simulink model "Main_Sim"  (R2018b)
settings: Solver=FixedStepAuto  StartTime=0.0  StopTime=10800  FixedStep=simParams.sample_time_s  RelTol=1e-3  EnableMultiTasking=on
values from neighbouring files (symbols this model uses):
  test_data = struct    [Sim_init.m]
undefined symbols (not defined in the file or in its folder): actuators_lib, Actuators_Lib, FSW_Lib, gyro_body_radps, gyro_meas_valid, mag_body_T, mag_meas_valid, photodiodes_A, simParams, solar_panel_power_W, sunsensor_body_deg, sunsensor_valid
libraries: gyroscope_lib x3, magnetometer_lib x3, dspstat3 x2, simulink_extras x2, rwa_assembly_torqueinput_lib x1, Environment_lib x1, allocation_lib x1, control_command_generation_lib x1, mode_select_lib x1, target_gen_lib x1, solar_panels_lib x1, sun_sensor_lib x1
settings Model: Creator=devantormey  LastModifiedBy=jeric
settings OptimizationCC: LifeSpan=inf
settings DebuggingCC: SFUnexpectedBacktrackingDiag=warning  SFNoUnconditionalDefaultTransitionDiag=warning
settings SFSimCC: SimUseLocalCustomCode=off
settings RTWCC: RTWUseLocalCustomCode=off
settings CodeAppCC: StateflowObjectComments=on
settings GRTTargetCC: TargetLangStandard=C89/C90 (ANSI)  GeneratePreprocessorConditionals=Disable all
settings ConfigComp: CovMetricSettings=dw  CovHtmlReporting=on  CovSaveCumulativeToWorkspaceVar=on  CovSaveSingleToWorkspaceVar=on  CovExternalEMLEnable=off

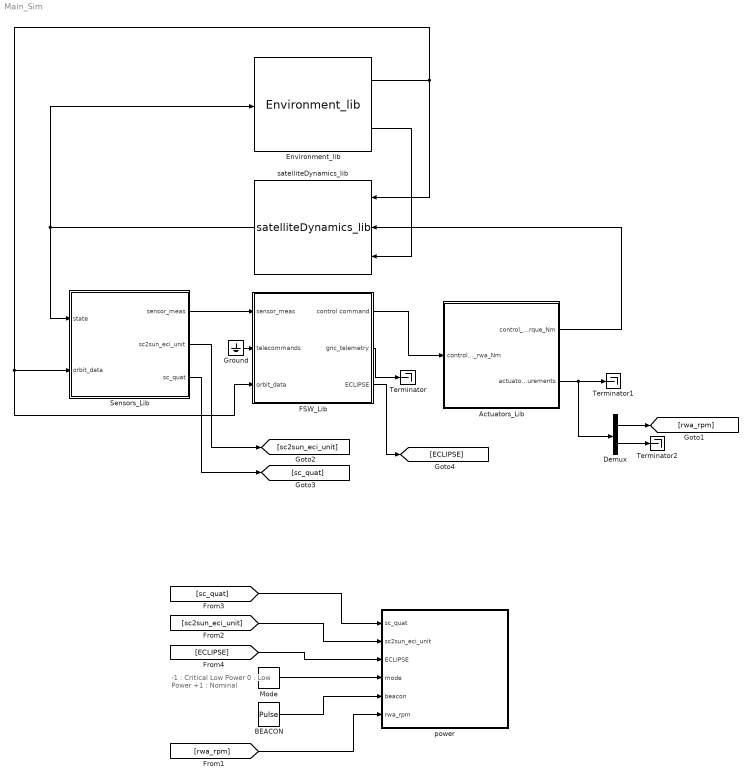
== system Main_Sim ==
  note: -1	: Critical Low Power
      |   0	: Low Power
      | +1	: Nominal
  Actuators_Lib : Subsystem  AncestorBlock=actuators_lib/Actuators_Lib
  BEACON : DiscretePulseGenerator  PulseType=Time based  Period=60  PulseWidth=100 * (1.0 / 60)
  Demux : Demux  Outputs=[4 4]
  Environment_lib : Environment_lib/Environment_lib  SystemSampleTime=-1
  FSW_Lib : Subsystem  AncestorBlock=FSW_Lib/FSW_Lib
  Ground : Ground
  Mode : Constant
  Sensors_Lib : Subsystem
  Terminator : Terminator
  Terminator1 : Terminator
  Terminator2 : Terminator
  power : Subsystem
  satelliteDynamics_lib : satelliteDynamics_lib/satelliteDynamics_lib  SystemSampleTime=-1
  wires:
  FSW_Lib/1(control command) -> Actuators_Lib/1(control_cmd_rwa_Nm)
  Sensors_Lib/1(sensor_meas) -> FSW_Lib/1(sensor_meas)
  satelliteDynamics_lib/1 -> Environment_lib/1, Sensors_Lib/1(state)
  Environment_lib/1 -> FSW_Lib/3(orbit_data), Sensors_Lib/2(orbit_data), satelliteDynamics_lib/1
  Environment_lib/2 -> satelliteDynamics_lib/3
  Actuators_Lib/1(control_torque_Nm) -> satelliteDynamics_lib/2
  Ground/1 -> FSW_Lib/2(telecommands)
  FSW_Lib/2(gnc_telemetry) -> Terminator/1
  Actuators_Lib/2(actuator_measurements) -> Demux/1, Terminator1/1
  Demux/1 -> [rwa_rpm]
  Demux/2 -> Terminator2/1
  Sensors_Lib/2(sc2sun_eci_unit) -> [sc2sun_eci_unit]
  Sensors_Lib/3(sc_quat) -> [sc_quat]
  FSW_Lib/3(ECLIPSE) -> [ECLIPSE]
  [sc2sun_eci_unit] -> power/2(sc2sun_eci_unit)
  [sc_quat] -> power/1(sc_quat)
  [ECLIPSE] -> power/3(ECLIPSE)
  Mode/1 -> power/4(mode)
  BEACON/1 -> power/5(beacon)
  [rwa_rpm] -> power/6(rwa_rpm)

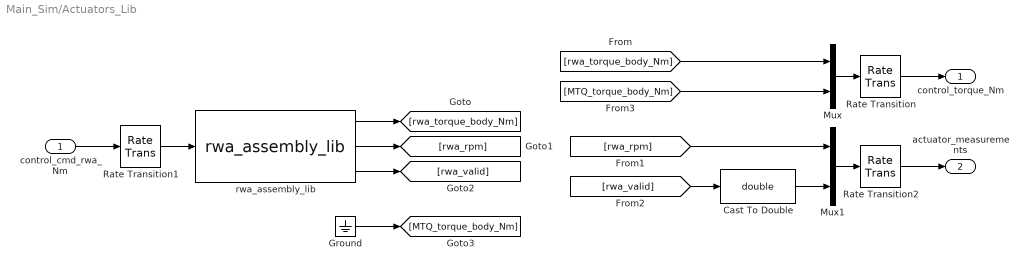
== system Main_Sim/Actuators_Lib ==
  control_cmd_rwa_Nm : Inport
  Cast To Double : DataTypeConversion  OutDataTypeStr=double
  Ground : Ground
  Mux : Mux  Inputs=[3 3]
  Mux1 : Mux  Inputs=[4 4]
  Rate Transition : RateTransition
  Rate Transition1 : RateTransition  OutPortSampleTimeOpt=Inherit  OutPortSampleTime=simParams.actuators.sample_time_s
  Rate Transition2 : RateTransition
  rwa_assembly_lib : rwa_assembly_torqueinput_lib/rwa_assembly_lib  SystemSampleTime=-1
  control_torque_Nm : Outport
  actuator_measurements : Outport  Port=2
  wires:
  Cast To Double/1 -> Mux1/2
  Rate Transition2/1 -> actuator_measurements/1
  Ground/1 -> [MTQ_torque_body_Nm]
  Mux/1 -> Rate Transition/1
  [rwa_torque_body_Nm] -> Mux/1
  [MTQ_torque_body_Nm] -> Mux/2
  Rate Transition1/1 -> rwa_assembly_lib/1
  Mux1/1 -> Rate Transition2/1
  [rwa_valid] -> Cast To Double/1
  [rwa_rpm] -> Mux1/1
  rwa_assembly_lib/1 -> [rwa_torque_body_Nm]
  rwa_assembly_lib/3 -> [rwa_valid]
  rwa_assembly_lib/2 -> [rwa_rpm]
  control_cmd_rwa_Nm/1 -> Rate Transition1/1
  Rate Transition/1 -> control_torque_Nm/1

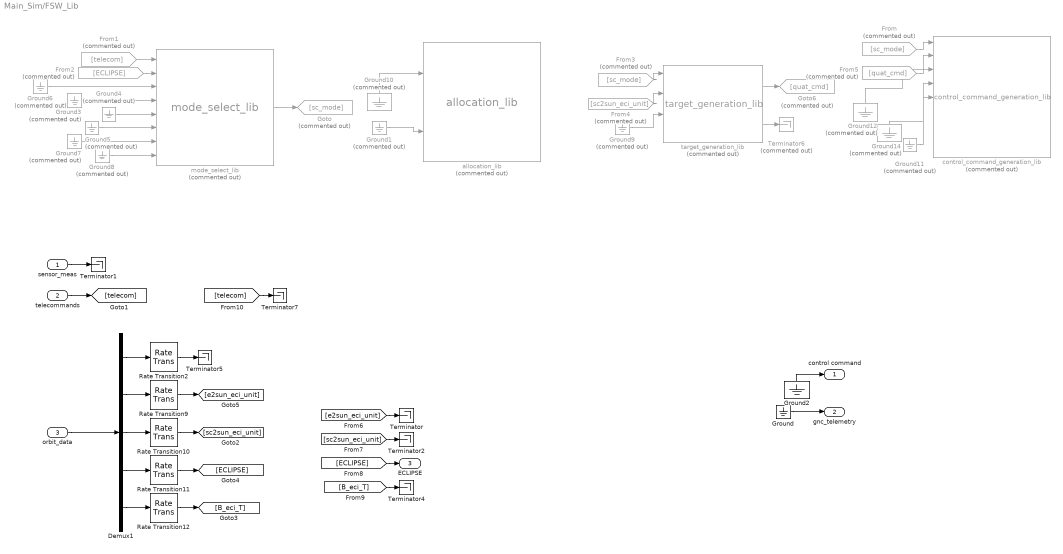
== system Main_Sim/FSW_Lib ==
  sensor_meas : Inport
  telecommands : Inport  Port=2
  orbit_data : Inport  Port=3
  Demux1 : Demux  Outputs=[3 3 3 1 3]
  From : From  Commented=on  GotoTag=sc_mode
  From1 : From  Commented=on  GotoTag=telecom
  From2 : From  Commented=on  GotoTag=ECLIPSE
  From3 : From  Commented=on  GotoTag=sc_mode
  From4 : From  Commented=on  GotoTag=sc2sun_eci_unit
  From5 : From  Commented=on  GotoTag=quat_cmd
  Goto : Goto  Commented=on  GotoTag=sc_mode
  Goto6 : Goto  Commented=on  GotoTag=quat_cmd
  Ground : Ground
  Ground{1,3..12,14} (12 alike) : Ground  Commented=on
  Ground2 : Ground
  Rate Transition{2,9..12} (5 alike) : RateTransition  OutPortSampleTime=simParams.sensors.sample_time_s
  Terminator{,1..2,4..5,7} (6 alike) : Terminator
  Terminator6 : Terminator  Commented=on
  allocation_lib : allocation_lib/allocation_lib  Commented=on  SystemSampleTime=-1
  control_command_generation_lib : control_command_generation_lib/control_command_generation_lib  Commented=on  SystemSampleTime=-1
  mode_select_lib : mode_select_lib/mode_select_lib  Commented=on  SystemSampleTime=-1
  target_generation_lib : target_gen_lib/target_generation_lib  Commented=on  SystemSampleTime=-1
  control command : Outport
  gnc_telemetry : Outport  Port=2
  ECLIPSE : Outport  Port=3
  wires:
  [telecom] -> Terminator7/1
  [B_eci_T] -> Terminator4/1
  [ECLIPSE] -> ECLIPSE/1
  [sc2sun_eci_unit] -> Terminator2/1
  [e2sun_eci_unit] -> Terminator/1
  Ground14/1 -> control_command_generation_lib/4
  Ground11/1 -> control_command_generation_lib/5
  Ground12/1 -> control_command_generation_lib/3
  Ground1/1 -> allocation_lib/2
  Ground10/1 -> allocation_lib/1
  From5/1 -> control_command_generation_lib/2
  Ground9/1 -> target_generation_lib/3
  target_generation_lib/1 -> Goto6/1
  target_generation_lib/2 -> Terminator6/1
  From4/1 -> target_generation_lib/2
  From3/1 -> target_generation_lib/1
  Ground8/1 -> mode_select_lib/8
  Ground7/1 -> mode_select_lib/7
  Ground6/1 -> mode_select_lib/3
  Ground5/1 -> mode_select_lib/6
  Ground4/1 -> mode_select_lib/5
  Ground3/1 -> mode_select_lib/4
  From2/1 -> mode_select_lib/2
  Demux1/4 -> Rate Transition11/1
  Rate Transition2/1 -> Terminator5/1
  Demux1/5 -> Rate Transition12/1
  Rate Transition9/1 -> [e2sun_eci_unit]
  Rate Transition10/1 -> [sc2sun_eci_unit]
  Demux1/3 -> Rate Transition10/1
  Rate Transition12/1 -> [B_eci_T]
  Demux1/1 -> Rate Transition2/1
  Rate Transition11/1 -> [ECLIPSE]
  Demux1/2 -> Rate Transition9/1
  orbit_data/1 -> Demux1/1
  From1/1 -> mode_select_lib/1
  From/1 -> control_command_generation_lib/1
  mode_select_lib/1 -> Goto/1
  Ground2/1 -> control command/1
  Ground/1 -> gnc_telemetry/1
  telecommands/1 -> [telecom]
  sensor_meas/1 -> Terminator1/1

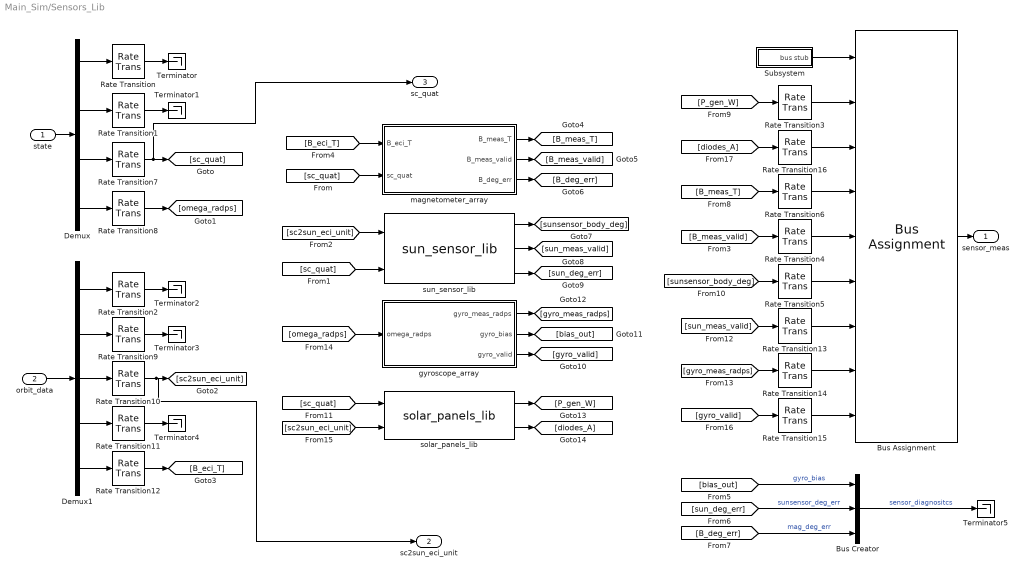
== system Main_Sim/Sensors_Lib ==
  state : Inport
  orbit_data : Inport  Port=2
  Bus Assignment : BusAssignment  AssignedSignals=solar_panel_power_W,photodiodes_A,mag_body_T,mag_meas_valid,sunsensor_body_deg,sunsensor_valid,gyro_body_radps,gyro_meas_valid
  Bus Creator : BusCreator  Inputs=3
  Demux : Demux  Outputs=[3 3 4 3]
  Demux1 : Demux  Outputs=[3 3 3 1 3]
  Rate Transition{,1..16} (17 alike) : RateTransition  OutPortSampleTime=simParams.sensors.sample_time_s
  Subsystem : Subsystem
  Terminator{,1..5} (6 alike) : Terminator
  gyroscope_array : Subsystem
  magnetometer_array : Subsystem
  solar_panels_lib : solar_panels_lib/solar_panels_lib  SystemSampleTime=-1
  "sun_sensor_lib " : sun_sensor_lib/sun_sensor_lib   SystemSampleTime=-1
  sensor_meas : Outport
  sc2sun_eci_unit : Outport  Port=2
  sc_quat : Outport  Port=3
  wires:
  [diodes_A] -> Rate Transition16/1
  Rate Transition16/1 -> Bus Assignment/3
  Rate Transition3/1 -> Bus Assignment/2
  Rate Transition6/1 -> Bus Assignment/4
  Rate Transition4/1 -> Bus Assignment/5
  Rate Transition5/1 -> Bus Assignment/6
  Rate Transition13/1 -> Bus Assignment/7
  Rate Transition14/1 -> Bus Assignment/8
  Rate Transition15/1 -> Bus Assignment/9
  solar_panels_lib/2 -> [diodes_A]
  Bus Creator/1 -> Terminator5/1  "sensor_diagnositcs"
  [B_deg_err] -> Bus Creator/3  "mag_deg_err"
  [sun_deg_err] -> Bus Creator/2  "sunsensor_deg_err"
  [bias_out] -> Bus Creator/1  "gyro_bias"
  [gyro_valid] -> Rate Transition15/1
  [gyro_meas_radps] -> Rate Transition14/1
  [sun_meas_valid] -> Rate Transition13/1
  [sunsensor_body_deg] -> Rate Transition5/1
  [B_meas_valid] -> Rate Transition4/1
  [P_gen_W] -> Rate Transition3/1
  [B_meas_T] -> Rate Transition6/1
  solar_panels_lib/1 -> [P_gen_W]
  [sc_quat] -> solar_panels_lib/1
  [sc2sun_eci_unit] -> solar_panels_lib/2
  Demux1/1 -> Rate Transition2/1
  Rate Transition2/1 -> Terminator2/1
  Rate Transition9/1 -> Terminator3/1
  Demux1/2 -> Rate Transition9/1
  Rate Transition10/1 -> sc2sun_eci_unit/1, [sc2sun_eci_unit]
  Demux1/3 -> Rate Transition10/1
  Rate Transition11/1 -> Terminator4/1
  Demux1/4 -> Rate Transition11/1
  Rate Transition12/1 -> [B_eci_T]
  Demux1/5 -> Rate Transition12/1
  Rate Transition/1 -> Terminator/1
  Demux/1 -> Rate Transition/1
  Rate Transition1/1 -> Terminator1/1
  Demux/2 -> Rate Transition1/1
  Rate Transition7/1 -> sc_quat/1, [sc_quat]
  Demux/3 -> Rate Transition7/1
  Demux/4 -> Rate Transition8/1
  Rate Transition8/1 -> [omega_radps]
  gyroscope_array/3(gyro_valid) -> [gyro_valid]
  gyroscope_array/2(gyro_bias) -> [bias_out]
  gyroscope_array/1(gyro_meas_radps) -> [gyro_meas_radps]
  "sun_sensor_lib "/3 -> [sun_deg_err]
  "sun_sensor_lib "/2 -> [sun_meas_valid]
  "sun_sensor_lib "/1 -> [sunsensor_body_deg]
  magnetometer_array/3(B_deg_err) -> [B_deg_err]
  magnetometer_array/2(B_meas_valid) -> [B_meas_valid]
  magnetometer_array/1(B_meas_T) -> [B_meas_T]
  Subsystem/1(bus stub) -> Bus Assignment/1
  [B_eci_T] -> magnetometer_array/1(B_eci_T)
  [sc2sun_eci_unit] -> "sun_sensor_lib "/1
  orbit_data/1 -> Demux1/1
  [omega_radps] -> gyroscope_array/1(omega_radps)
  [sc_quat] -> "sun_sensor_lib "/2
  [sc_quat] -> magnetometer_array/2(sc_quat)
  state/1 -> Demux/1
  Bus Assignment/1 -> sensor_meas/1

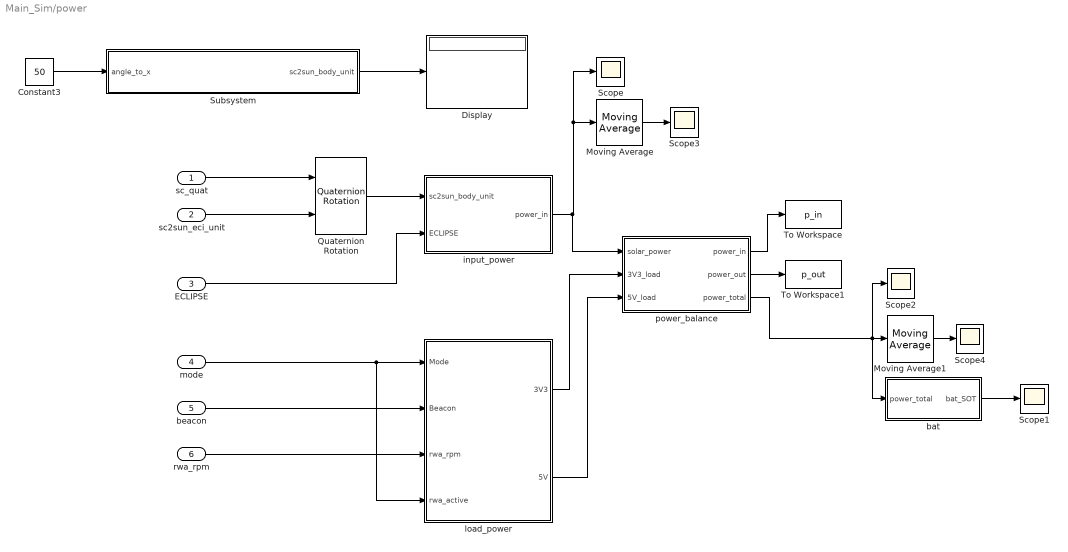
== system Main_Sim/power ==
  sc_quat : Inport
  sc2sun_eci_unit : Inport  Port=2
  ECLIPSE : Inport  Port=3
  mode : Inport  Port=4
  beacon : Inport  Port=5
  rwa_rpm : Inport  Port=6
  Constant3 : Constant  Value=50
  Display : Display
  Moving Average : dspstat3/Moving Average  Method=Exponential weighting  ForgettingFactorPort=off  SpecifyWindowLength=on  WindowLength=4  ForgettingFactor=1.0  SimulateUsing=Code generation
  Moving Average1 : dspstat3/Moving Average  Method=Exponential weighting  ForgettingFactorPort=off  SpecifyWindowLength=on  WindowLength=4  ForgettingFactor=1.0  SimulateUsing=Code generation
  Quaternion Rotation : aerolibutil/Quaternion Rotation
  Scope{,1..4} (5 alike) : Scope
  Subsystem : Subsystem
  To Workspace : ToWorkspace  VariableName=p_in  SampleTime=-1
  To Workspace1 : ToWorkspace  VariableName=p_out  SampleTime=-1
  bat : Subsystem
  input_power : Subsystem
  load_power : Subsystem
  power_balance : Subsystem
  wires:
  load_power/1(3V3) -> power_balance/2("3V3_load ")
  input_power/1(power_in) -> power_balance/1(solar_power), Moving Average/1, Scope/1
  rwa_rpm/1 -> load_power/3(rwa_rpm)
  mode/1 -> load_power/4(rwa_active), load_power/1(Mode)
  beacon/1 -> load_power/2(Beacon)
  Moving Average1/1 -> Scope4/1
  load_power/2(5V) -> power_balance/3(5V_load)
  bat/1(bat_SOT) -> Scope1/1
  Moving Average/1 -> Scope3/1
  sc_quat/1 -> Quaternion Rotation/1
  sc2sun_eci_unit/1 -> Quaternion Rotation/2
  ECLIPSE/1 -> input_power/2(ECLIPSE)
  power_balance/3(power_total) -> Scope2/1, bat/1(power_total), Moving Average1/1
  power_balance/1(power_in) -> To Workspace/1
  power_balance/2(power_out) -> To Workspace1/1
  Constant3/1 -> Subsystem/1(angle_to_x)
  Subsystem/1(sc2sun_body_unit) -> Display/1
  Quaternion Rotation/1 -> input_power/1(sc2sun_body_unit)

== system Main_Sim/Sensors_Lib/Subsystem ==
  Bus Creator : BusCreator  Inputs=8
  Constant : Constant  Value=zeros(6, 1)
  Constant1 : Constant  Value=zeros(3, simParams.sensors.mag.N_mag)
  Constant2 : Constant  Value=zeros(2, 1)
  Constant3 : Constant  Value=zeros(3, simParams.sensors.gyro.N_gyro)
  Constant4 : Constant  Value=zeros(1,simParams.sensors.mag.N_mag)
  Constant5 : Constant  Value=0
  Constant6 : Constant  Value=zeros(1,simParams.sensors.gyro.N_gyro)
  Constant7 : Constant  Value=zeros(6, 1)
  bus stub : Outport
  wires:
  Constant7/1 -> Bus Creator/2  "photodiodes_A"
  Constant6/1 -> Bus Creator/8  "gyro_meas_valid"
  Constant5/1 -> Bus Creator/6  "sunsensor_valid"
  Constant4/1 -> Bus Creator/4  "mag_meas_valid"
  Constant3/1 -> Bus Creator/7  "gyro_body_radps"
  Bus Creator/1 -> bus stub/1
  Constant2/1 -> Bus Creator/5  "sunsensor_body_deg"
  Constant1/1 -> Bus Creator/3  "mag_body_T"
  Constant/1 -> Bus Creator/1  "solar_panel_power_W"

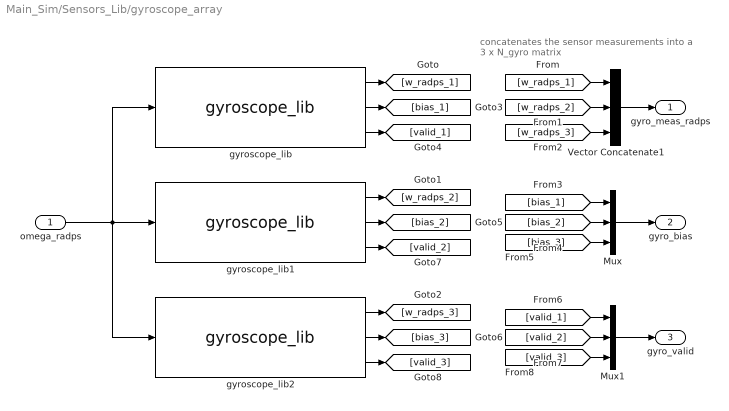
== system Main_Sim/Sensors_Lib/gyroscope_array ==
  note: concatenates the sensor measurements
      | into a 3 x N_gyro matrix
  omega_radps : Inport
  Mux : Mux  Inputs=3
  Mux1 : Mux  Inputs=3
  Vector Concatenate1 : Concatenate  NumInputs=3  Mode=Multidimensional array  ConcatenateDimension=2
  gyroscope_lib : gyroscope_lib/gyroscope_lib  id_s=1
  gyroscope_lib1 : gyroscope_lib/gyroscope_lib  id_s=2
  gyroscope_lib2 : gyroscope_lib/gyroscope_lib  id_s=3
  gyro_meas_radps : Outport
  gyro_bias : Outport  Port=2
  gyro_valid : Outport  Port=3
  wires:
  [valid_3] -> Mux1/3
  [valid_2] -> Mux1/2
  [valid_1] -> Mux1/1
  Mux1/1 -> gyro_valid/1
  [bias_3] -> Mux/3
  [bias_2] -> Mux/2
  [bias_1] -> Mux/1
  Mux/1 -> gyro_bias/1
  [w_radps_3] -> Vector Concatenate1/3
  [w_radps_2] -> Vector Concatenate1/2
  [w_radps_1] -> Vector Concatenate1/1
  Vector Concatenate1/1 -> gyro_meas_radps/1
  gyroscope_lib2/3 -> [valid_3]
  gyroscope_lib1/3 -> [valid_2]
  gyroscope_lib2/2 -> [bias_3]
  gyroscope_lib1/2 -> [bias_2]
  gyroscope_lib/3 -> [valid_1]
  gyroscope_lib/2 -> [bias_1]
  gyroscope_lib2/1 -> [w_radps_3]
  gyroscope_lib1/1 -> [w_radps_2]
  gyroscope_lib/1 -> [w_radps_1]
  omega_radps/1 -> gyroscope_lib1/1, gyroscope_lib/1, gyroscope_lib2/1

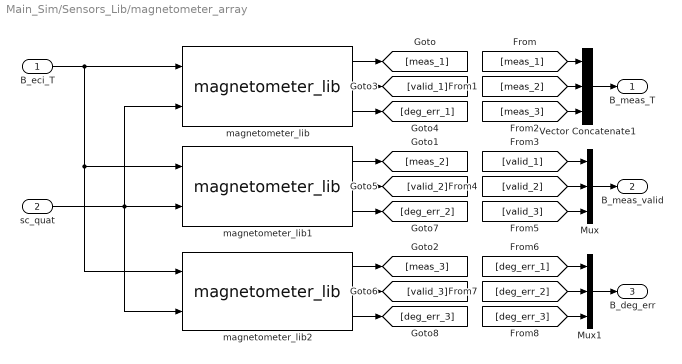
== system Main_Sim/Sensors_Lib/magnetometer_array ==
  B_eci_T : Inport
  sc_quat : Inport  Port=2
  Mux : Mux  Inputs=3
  Mux1 : Mux  Inputs=3
  Vector Concatenate1 : Concatenate  NumInputs=3  Mode=Multidimensional array  ConcatenateDimension=2
  magnetometer_lib : magnetometer_lib/magnetometer_lib  id_s=1
  magnetometer_lib1 : magnetometer_lib/magnetometer_lib  id_s=2
  magnetometer_lib2 : magnetometer_lib/magnetometer_lib  id_s=1
  B_meas_T : Outport
  B_meas_valid : Outport  Port=2
  B_deg_err : Outport  Port=3
  wires:
  [deg_err_3] -> Mux1/3
  [deg_err_2] -> Mux1/2
  [deg_err_1] -> Mux1/1
  Mux1/1 -> B_deg_err/1
  [valid_3] -> Mux/3
  [valid_2] -> Mux/2
  [valid_1] -> Mux/1
  Mux/1 -> B_meas_valid/1
  [meas_3] -> Vector Concatenate1/3
  [meas_2] -> Vector Concatenate1/2
  [meas_1] -> Vector Concatenate1/1
  Vector Concatenate1/1 -> B_meas_T/1
  magnetometer_lib2/3 -> [deg_err_3]
  magnetometer_lib1/3 -> [deg_err_2]
  magnetometer_lib2/2 -> [valid_3]
  magnetometer_lib1/2 -> [valid_2]
  magnetometer_lib/3 -> [deg_err_1]
  magnetometer_lib/2 -> [valid_1]
  magnetometer_lib2/1 -> [meas_3]
  magnetometer_lib1/1 -> [meas_2]
  magnetometer_lib/1 -> [meas_1]
  B_eci_T/1 -> magnetometer_lib1/1, magnetometer_lib2/1, magnetometer_lib/1
  sc_quat/1 -> magnetometer_lib1/2, magnetometer_lib2/2, magnetometer_lib/2

== system Main_Sim/power/Subsystem ==
  angle_to_x : Inport
  Constant1 : Constant  Value=90
  Constant2 : Constant  Value=0
  Cos : Trigonometry  Operator=cos
  Cos1 : Trigonometry  Operator=cos
  Degrees to Radians : simulink_extras/Transformations/Degrees to Radians
  Degrees to Radians1 : simulink_extras/Transformations/Degrees to Radians
  Mux : Mux  Inputs=3
  Subtract : Sum  Inputs=+-
  sc2sun_body_unit : Outport
  wires:
  Subtract/1 -> Degrees to Radians1/1
  Constant2/1 -> Mux/3
  Cos1/1 -> Mux/2
  Degrees to Radians1/1 -> Cos1/1
  Degrees to Radians/1 -> Cos/1
  Cos/1 -> Mux/1
  Mux/1 -> sc2sun_body_unit/1
  Constant1/1 -> Subtract/1
  angle_to_x/1 -> Subtract/2, Degrees to Radians/1

== system Main_Sim/power/bat ==
  power_total : Inport
  Constant4 : Constant  Value=1/(60*60)
  Constant5 : Constant  Value=20000
  Divide : Product  Inputs=*/
  Integrator : Integrator  InitialCondition=20000  LimitOutput=on  UpperSaturationLimit=20000  LowerSaturationLimit=0
  Product : Product
  bat_SOT : Outport
  wires:
  Constant4/1 -> Product/2
  Constant5/1 -> Divide/2
  power_total/1 -> Product/1
  Product/1 -> Integrator/1
  Integrator/1 -> Divide/1
  Divide/1 -> bat_SOT/1

== system Main_Sim/power/input_power ==
  sc2sun_body_unit : Inport
  ECLIPSE : Inport  Port=2
  Constant1 : Constant
  Product : Product
  Subtract : Sum  Inputs=+-
  Sum of Elements : Sum  Inputs=+
  Terminator : Terminator
  solar_panel_power : MATLAB Function  TreatAsAtomicUnit=on
  power_in : Outport
  wires:
  Product/1 -> Sum of Elements/1
  solar_panel_power/2(diodes_A) -> Terminator/1
  solar_panel_power/1(power_gen_W) -> Product/1
  Sum of Elements/1 -> power_in/1
  sc2sun_body_unit/1 -> solar_panel_power/1(sc2sun_body_unit)
  Constant1/1 -> Subtract/1
  ECLIPSE/1 -> Subtract/2
  Subtract/1 -> Product/2

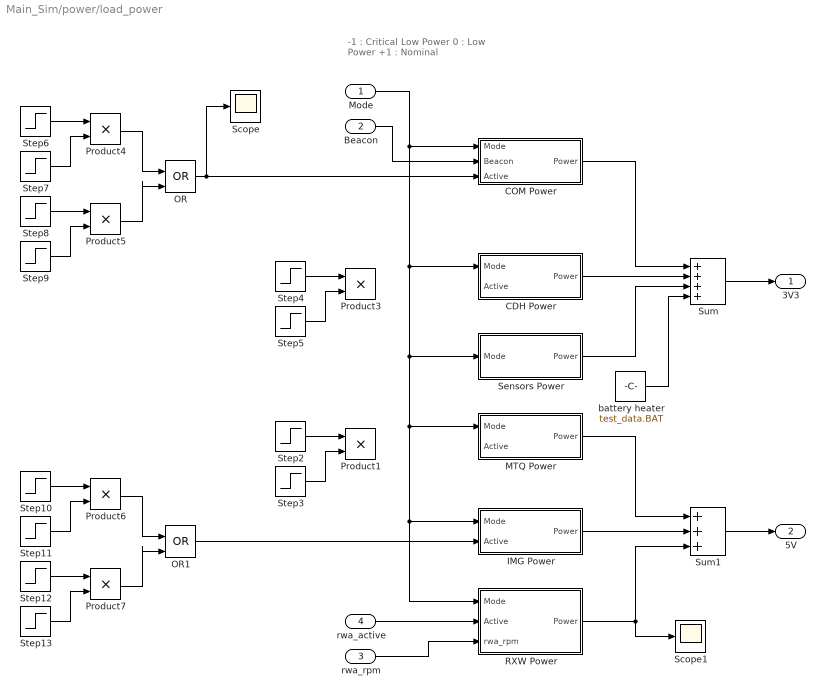
== system Main_Sim/power/load_power ==
  note: -1	: Critical Low Power
      |   0	: Low Power
      | +1	: Nominal
  Mode : Inport
  Beacon : Inport  Port=2
  rwa_rpm : Inport  Port=3
  rwa_active : Inport  Port=4
  CDH Power : Subsystem
  COM Power : Subsystem
  IMG Power : Subsystem
  MTQ Power : Subsystem
  OR : Logic  Operator=OR  IconShape=distinctive  AllPortsSameDT=off  OutDataTypeStr=boolean
  OR1 : Logic  Operator=OR  IconShape=distinctive  AllPortsSameDT=off  OutDataTypeStr=boolean
  Product{1,3..7} (6 alike) : Product
  RXW Power : Subsystem
  Scope : Scope
  Scope1 : Scope
  Sensors Power : Subsystem
  Step10 : Step  Time=2000  SampleTime=0
  Step11 : Step  Time=2300  Before=1  After=0  SampleTime=0
  Step12 : Step  Time=7400  SampleTime=0
  Step13 : Step  Time=7700  Before=1  After=0  SampleTime=0
  Step2 : Step  Time=2000  SampleTime=0
  Step3 : Step  Time=3800  Before=1  After=0  SampleTime=0
  Step4 : Step  Time=3500  SampleTime=0
  Step5 : Step  Time=3800  Before=1  After=0  SampleTime=0
  Step6 : Step  Time=2000  SampleTime=0
  Step7 : Step  Time=2300  Before=1  After=0  SampleTime=0
  Step8 : Step  Time=7400  SampleTime=0
  Step9 : Step  Time=7700  Before=1  After=0  SampleTime=0
  Sum : Sum  Inputs=++++
  Sum1 : Sum  Inputs=+++
  battery heater : Constant  Value=test_data.BAT
  3V3 : Outport
  5V : Outport  Port=2
  wires:
  Mode/1 -> RXW Power/1(Mode), IMG Power/1(Mode), MTQ Power/1(Mode), Sensors Power/1(Mode), CDH Power/1(Mode), COM Power/1(Mode)
  Beacon/1 -> COM Power/2(Beacon)
  rwa_active/1 -> RXW Power/2(Active)
  CDH Power/1(Power) -> Sum/2
  COM Power/1(Power) -> Sum/1
  Sensors Power/1(Power) -> Sum/3
  IMG Power/1(Power) -> Sum1/2
  RXW Power/1(Power) -> Scope1/1, Sum1/3
  Sum/1 -> 3V3/1
  Sum1/1 -> 5V/1
  battery heater/1 -> Sum/4
  rwa_rpm/1 -> RXW Power/3(rwa_rpm)
  Step3/1 -> Product1/2
  Step2/1 -> Product1/1
  Step4/1 -> Product3/1
  Step5/1 -> Product3/2
  Step7/1 -> Product4/2
  Step6/1 -> Product4/1
  MTQ Power/1(Power) -> Sum1/1
  Step9/1 -> Product5/2
  Step8/1 -> Product5/1
  Product4/1 -> OR/1
  Product5/1 -> OR/2
  OR/1 -> COM Power/3("Active "), Scope/1
  OR1/1 -> IMG Power/2(Active)
  Step12/1 -> Product7/1
  Product7/1 -> OR1/2
  Step13/1 -> Product7/2
  Step11/1 -> Product6/2
  Product6/1 -> OR1/1
  Step10/1 -> Product6/1

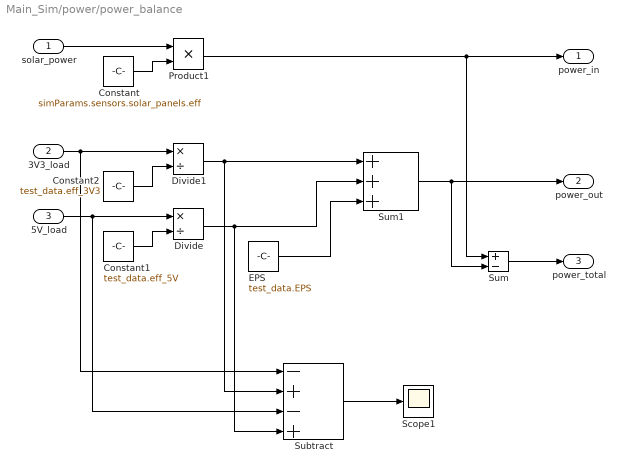
== system Main_Sim/power/power_balance ==
  solar_power : Inport
  "3V3_load " : Inport  Port=2
  5V_load : Inport  Port=3
  Constant : Constant  Value=simParams.sensors.solar_panels.eff
  Constant1 : Constant  Value=test_data.eff_5V
  Constant2 : Constant  Value=test_data.eff_3V3
  Divide : Product  Inputs=*/
  Divide1 : Product  Inputs=*/
  EPS : Constant  Value=test_data.EPS
  Product1 : Product
  Scope1 : Scope
  Subtract : Sum  Inputs=-+-+
  Sum : Sum  Inputs=+-
  Sum1 : Sum  Inputs=+++
  power_in : Outport
  power_out : Outport  Port=2
  power_total : Outport  Port=3
  wires:
  solar_power/1 -> Product1/1
  Constant/1 -> Product1/2
  5V_load/1 -> Subtract/3, Divide/1
  Constant1/1 -> Divide/2
  Constant2/1 -> Divide1/2
  "3V3_load "/1 -> Subtract/1, Divide1/1
  Divide1/1 -> Sum1/1, Subtract/2
  Product1/1 -> Sum/1, power_in/1
  Divide/1 -> Sum1/2, Subtract/4
  Sum1/1 -> Sum/2, power_out/1
  EPS/1 -> Sum1/3
  Subtract/1 -> Scope1/1
  Sum/1 -> power_total/1

== system Main_Sim/power/load_power/CDH Power ==
  Mode : Inport
  Active : Inport  Port=2
  Constant : Constant  Value=-1
  Constant1 : Constant  Value=test_data.CDH_Idle
  Constant2 : Constant  Value=test_data.CDH_Active
  GreaterThan : RelationalOperator  OutDataTypeStr=boolean  RndMeth=Simplest
  Logical Operator : Logic  AllPortsSameDT=off  OutDataTypeStr=boolean
  Switch : Switch  Criteria=u2 > Threshold
  Power : Outport  VectorParamsAs1DForOutWhenUnconnected=on
  wires:
  Constant/1 -> GreaterThan/2
  Mode/1 -> GreaterThan/1
  GreaterThan/1 -> Logical Operator/1
  Active/1 -> Logical Operator/2
  Logical Operator/1 -> Switch/2
  Switch/1 -> Power/1
  Constant2/1 -> Switch/1
  Constant1/1 -> Switch/3

== system Main_Sim/power/load_power/COM Power ==
  Mode : Inport
  Beacon : Inport  Port=2
  "Active " : Inport  Port=3
  Constant : Constant  Value=0
  Constant1 : Constant  Value=test_data.COM_RX
  Constant2 : Constant  Value=test_data.COM_TX+test_data.COM_RX
  GreaterThan : RelationalOperator  OutDataTypeStr=boolean  RndMeth=Simplest
  Logical Operator : Logic  AllPortsSameDT=off  OutDataTypeStr=boolean
  OR : Logic  Operator=OR  IconShape=distinctive  AllPortsSameDT=off  OutDataTypeStr=boolean
  Switch : Switch  Criteria=u2 > Threshold
  Power : Outport  VectorParamsAs1DForOutWhenUnconnected=on
  wires:
  Constant/1 -> GreaterThan/2
  Mode/1 -> GreaterThan/1
  GreaterThan/1 -> Logical Operator/1
  Constant2/1 -> Switch/1
  Constant1/1 -> Switch/3
  Logical Operator/1 -> Switch/2
  Switch/1 -> Power/1
  Beacon/1 -> OR/1
  "Active "/1 -> OR/2
  OR/1 -> Logical Operator/2

== system Main_Sim/power/load_power/IMG Power ==
  Mode : Inport
  Active : Inport  Port=2
  Constant : Constant
  Constant1 : Constant  Value=test_data.IMG_Idle
  Constant2 : Constant  Value=test_data.IMG_Active
  GreaterThan : RelationalOperator  OutDataTypeStr=boolean  RndMeth=Simplest
  Logical Operator : Logic  AllPortsSameDT=off  OutDataTypeStr=boolean
  Switch : Switch  Criteria=u2 > Threshold
  Power : Outport  VectorParamsAs1DForOutWhenUnconnected=on
  wires:
  Constant/1 -> GreaterThan/2
  Mode/1 -> GreaterThan/1
  GreaterThan/1 -> Logical Operator/1
  Active/1 -> Logical Operator/2
  Logical Operator/1 -> Switch/2
  Constant2/1 -> Switch/1
  Constant1/1 -> Switch/3
  Switch/1 -> Power/1

== system Main_Sim/power/load_power/MTQ Power ==
  Mode : Inport
  Active : Inport  Port=2
  Constant : Constant
  Constant1 : Constant  Value=test_data.MTQ_Active
  Constant2 : Constant  Value=test_data.MTQ_Idle
  GreaterThan : RelationalOperator  OutDataTypeStr=boolean  RndMeth=Simplest
  Logical Operator : Logic  AllPortsSameDT=off  OutDataTypeStr=boolean
  Switch : Switch  Criteria=u2 > Threshold
  Power : Outport  VectorParamsAs1DForOutWhenUnconnected=on
  wires:
  Constant/1 -> GreaterThan/2
  Mode/1 -> GreaterThan/1
  GreaterThan/1 -> Logical Operator/1
  Constant1/1 -> Switch/1
  Active/1 -> Logical Operator/2
  Logical Operator/1 -> Switch/2
  Constant2/1 -> Switch/3
  Switch/1 -> Power/1

== system Main_Sim/power/load_power/RXW Power ==
  Mode : Inport
  Active : Inport  Port=2
  rwa_rpm : Inport  Port=3
  Subsystem1 : Subsystem
  Power : Outport  VectorParamsAs1DForOutWhenUnconnected=on
  wires:
  Mode/1 -> Subsystem1/1(Mode)
  Active/1 -> Subsystem1/2(Active)
  rwa_rpm/1 -> Subsystem1/3(RPM)
  Subsystem1/1(Power) -> Power/1

== system Main_Sim/power/load_power/Sensors Power ==
  Mode : Inport
  Constant : Constant  Value=0
  Constant1 : Constant  Value=test_data.SEN_AVG
  GreaterThan : RelationalOperator  OutDataTypeStr=boolean  RndMeth=Simplest
  Product1 : Product
  Power : Outport  VectorParamsAs1DForOutWhenUnconnected=on
  wires:
  Constant/1 -> GreaterThan/2
  Mode/1 -> GreaterThan/1
  GreaterThan/1 -> Product1/2
  Constant1/1 -> Product1/1
  Product1/1 -> Power/1

== system Main_Sim/power/load_power/RXW Power/Subsystem1 ==
  Mode : Inport
  Active : Inport  Port=2
  RPM : Inport  Port=3
  Demux : Demux
  Subsystem : Subsystem
  Subsystem1 : Subsystem
  Subsystem2 : Subsystem
  Subsystem3 : Subsystem
  Sum : Sum  Inputs=++++
  Power : Outport
  wires:
  RPM/1 -> Demux/1
  Mode/1 -> Subsystem3/1(Mode), Subsystem2/1(Mode), Subsystem1/1(Mode), Subsystem/1(Mode)
  Active/1 -> Subsystem3/2(Active), Subsystem2/2(Active), Subsystem1/2(Active), Subsystem/2(Active)
  Demux/1 -> Subsystem/3(RPM)
  Demux/2 -> Subsystem1/3(RPM)
  Demux/3 -> Subsystem2/3(RPM)
  Demux/4 -> Subsystem3/3(RPM)
  Subsystem1/1(Power) -> Sum/2
  Subsystem2/1(Power) -> Sum/3
  Subsystem3/1(Power) -> Sum/4
  Subsystem/1(Power) -> Sum/1
  Sum/1 -> Power/1

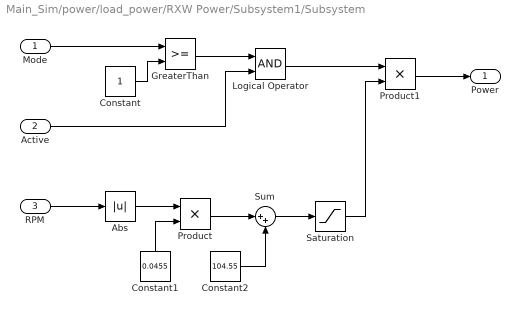
== system Main_Sim/power/load_power/RXW Power/Subsystem1/Subsystem ==
  Mode : Inport
  Active : Inport  Port=2
  RPM : Inport  Port=3
  Abs : Abs
  Constant : Constant
  Constant1 : Constant  Value=0.0455
  Constant2 : Constant  Value=104.55
  GreaterThan : RelationalOperator  OutDataTypeStr=boolean  RndMeth=Simplest
  Logical Operator : Logic  AllPortsSameDT=off  OutDataTypeStr=boolean
  Product : Product
  Product1 : Product
  Saturation : Saturate  UpperLimit=inf  LowerLimit=150
  Sum : Sum  Inputs=|++
  Power : Outport
  wires:
  Constant1/1 -> Product/2
  Logical Operator/1 -> Product1/1
  GreaterThan/1 -> Logical Operator/1
  Mode/1 -> GreaterThan/1
  Active/1 -> Logical Operator/2
  Constant/1 -> GreaterThan/2
  Product/1 -> Sum/1
  Constant2/1 -> Sum/2
  Sum/1 -> Saturation/1
  RPM/1 -> Abs/1
  Abs/1 -> Product/1
  Saturation/1 -> Product1/2
  Product1/1 -> Power/1

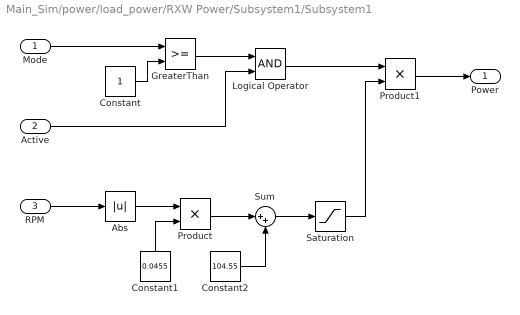
== system Main_Sim/power/load_power/RXW Power/Subsystem1/Subsystem1 ==
  Mode : Inport
  Active : Inport  Port=2
  RPM : Inport  Port=3
  Abs : Abs
  Constant : Constant
  Constant1 : Constant  Value=0.0455
  Constant2 : Constant  Value=104.55
  GreaterThan : RelationalOperator  OutDataTypeStr=boolean  RndMeth=Simplest
  Logical Operator : Logic  AllPortsSameDT=off  OutDataTypeStr=boolean
  Product : Product
  Product1 : Product
  Saturation : Saturate  UpperLimit=inf  LowerLimit=150
  Sum : Sum  Inputs=|++
  Power : Outport
  wires:
  Constant1/1 -> Product/2
  Logical Operator/1 -> Product1/1
  GreaterThan/1 -> Logical Operator/1
  Mode/1 -> GreaterThan/1
  Active/1 -> Logical Operator/2
  Constant/1 -> GreaterThan/2
  Product/1 -> Sum/1
  Constant2/1 -> Sum/2
  Sum/1 -> Saturation/1
  RPM/1 -> Abs/1
  Abs/1 -> Product/1
  Saturation/1 -> Product1/2
  Product1/1 -> Power/1

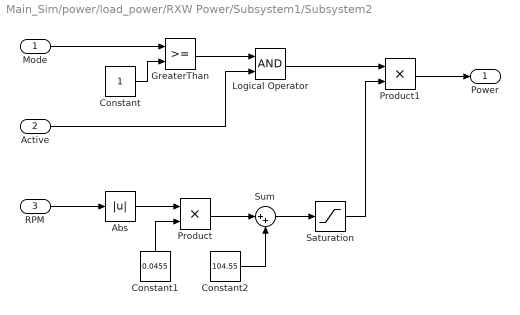
== system Main_Sim/power/load_power/RXW Power/Subsystem1/Subsystem2 ==
  Mode : Inport
  Active : Inport  Port=2
  RPM : Inport  Port=3
  Abs : Abs
  Constant : Constant
  Constant1 : Constant  Value=0.0455
  Constant2 : Constant  Value=104.55
  GreaterThan : RelationalOperator  OutDataTypeStr=boolean  RndMeth=Simplest
  Logical Operator : Logic  AllPortsSameDT=off  OutDataTypeStr=boolean
  Product : Product
  Product1 : Product
  Saturation : Saturate  UpperLimit=inf  LowerLimit=150
  Sum : Sum  Inputs=|++
  Power : Outport
  wires:
  Constant1/1 -> Product/2
  Logical Operator/1 -> Product1/1
  GreaterThan/1 -> Logical Operator/1
  Mode/1 -> GreaterThan/1
  Active/1 -> Logical Operator/2
  Constant/1 -> GreaterThan/2
  Product/1 -> Sum/1
  Constant2/1 -> Sum/2
  Sum/1 -> Saturation/1
  RPM/1 -> Abs/1
  Abs/1 -> Product/1
  Saturation/1 -> Product1/2
  Product1/1 -> Power/1

== system Main_Sim/power/load_power/RXW Power/Subsystem1/Subsystem3 ==
  Mode : Inport
  Active : Inport  Port=2
  RPM : Inport  Port=3
  Abs : Abs
  Constant : Constant
  Constant1 : Constant  Value=0.0455
  Constant2 : Constant  Value=104.55
  GreaterThan : RelationalOperator  OutDataTypeStr=boolean  RndMeth=Simplest
  Logical Operator : Logic  AllPortsSameDT=off  OutDataTypeStr=boolean
  Product : Product
  Product1 : Product
  Saturation : Saturate  UpperLimit=inf  LowerLimit=150
  Sum : Sum  Inputs=|++
  Power : Outport
  wires:
  Constant1/1 -> Product/2
  Logical Operator/1 -> Product1/1
  GreaterThan/1 -> Logical Operator/1
  Mode/1 -> GreaterThan/1
  Active/1 -> Logical Operator/2
  Constant/1 -> GreaterThan/2
  Product/1 -> Sum/1
  Constant2/1 -> Sum/2
  Sum/1 -> Saturation/1
  RPM/1 -> Abs/1
  Abs/1 -> Product/1
  Saturation/1 -> Product1/2
  Product1/1 -> Power/1

== matlab function Main_Sim/power/input_power/solar_panel_power ==
  data: sc2sun_body_unit input; power_gen_W output; simParams parameter; diodes_A output
function [power_gen_W,diodes_A] = get_power_gen(sc2sun_body_unit,simParams)
%GET_POWER_GEN
% 
% get_power_gen(sc2sun_body_unit,simParams) computes the total power being
% generated by the solar panels located on each of face. Assumes power
% generation is proportional to the square of the cosine of the incidence 
% angle to the sun, and can generate a maximum of 'maxPower' for each face.
%
% Assumes there are solar panels on all 6 sides of cuboid s/c, but fewer
% faces can be modeled by setting the 'maxPower' of those faces to zero.
% ORDER OF FACES: [ +x, -x, +y, -y, +z, -z ]
%
% This function also outputs the current reading from the photodiode on
% each face in Amps as diodes_A
%
% T. Reynolds
%#codegen

power_gen_W = zeros(6,1);
diodes_A    = zeros(6,1);
normals     = simParams.sensors.solar_panels.normals;
maxPower    = simParams.sensors.solar_panels.maxPower;
I_out_ApW   = simParams.sensors.photodiodes.I_out_ApW;

for k = 1:6
   % compute cos(incidence)
   sdotf = dot(normals(:,k),sc2sun_body_unit);
   cinc  = saturate(sdotf);
   incidence = acos(cinc);
   
   if incidence > 0.698132 % greater than 40 degrees
       factor = (-0.369 * cinc^3) + (0.637 * cinc^2) + (0.75 * cinc) -0.015;
   else
       factor = cinc;
   end
       
   if factor < 0
       factor = 0;
   end
   % compute power generated on ith face
   power_gen_W(k) = maxPower(k) * factor; %* cinc * cinc;
   
   % compute photodiode current
   diodes_A(k) = power_gen_W(k) * I_out_ApW; 
end

end

function y = saturate(x)
    if( x < 0 )
        y = 0.0;
    elseif( x >= 1.0 )
        y = 1.0;
    else
        y = x;
    end
end
